simulink model "summer21"  (R2021a)
settings: Solver=VariableStepAuto  StartTime=0.0  StopTime=15  RelTol=1e-3
values from neighbouring files (symbols this model uses):
  C = num{1}(2:end)    [MR2007_final_P1_vt17.m]    (also in MR2007_final_fall17.m = [1, 0]; MR2007_final_p2.m = [1, 0]; MR2007_summer2021.m = B; map.m = [1, 0])
  Gamma = [1;0]    [MR2007_final_P1_vt17.m]    (also in MR2007_final_fall17.m = [1/omega0^2*(cosh(omega0*h) - 1); 1/omega0*sinh(omega0*h)]; MR2007_final_p2.m = [0.5;1]; MR2007_summer2021.m)
  l0 = 1/dcgain(sys_c)    [MR2007_summer2021.m]
  L_e = acker(Phi_e, Gamma_e, [pc, 0.5])    [MR2007_summer2021.m]
  Phi = cat(1, -den{1}(2:end), [1, 0])    [MR2007_final_P1_vt17.m]    (also in MR2007_final_fall17.m = [cosh(omega0*h), 1/omega0*sinh(omega0*h); MR2007_final_p2.m = [1 1; 0 1]; MR2007_summer2021.m = [-A(2:end); 1 0])
settings Model: Creator=kjartan  LastModifiedBy=kjartan

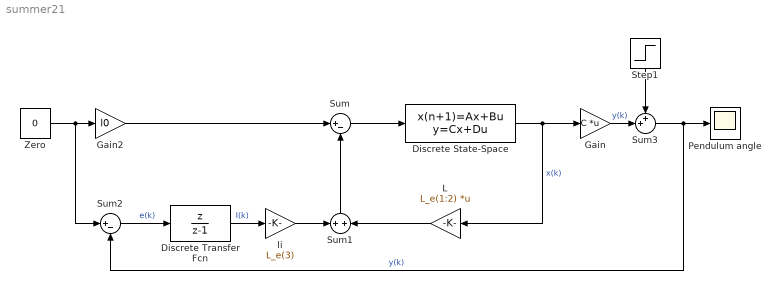
== system summer21 ==
  Discrete Transfer Fcn : DiscreteTransferFcn  Numerator=[1, 0]  Denominator=[1 -1]
  Discrete State-Space : DiscreteStateSpace  A=Phi  B=Gamma  C=eye(2)  D=zeros(2,1)  SampleTime=-1
  Gain : Gain  Gain=C  Multiplication=Matrix(K*u) (u vector)
  Gain2 : Gain  Gain=l0
  L : Gain  Gain=L_e(1:2)  Multiplication=Matrix(K*u) (u vector)
  Pendulum angle : Scope
  Step1 : Step  SampleTime=0
  Sum : Sum  Inputs=|+-
  Sum1 : Sum  Inputs=+|+
  Sum2 : Sum  Inputs=|+-
  Sum3 : Sum  Inputs=++|
  Zero : Constant  Value=0  OutDataTypeStr=Inherit: Inherit via back propagation
  li : Gain  Gain=L_e(3)
  wires:
  Discrete State-Space/1 -> L/1, Gain/1  "x(k)"
  Sum3/1 -> Sum2/2, Pendulum angle/1  "y(k)"
  Sum1/1 -> Sum/2
  L/1 -> Sum1/2
  Zero/1 -> Sum2/1, Gain2/1
  Sum2/1 -> Discrete Transfer Fcn/1  "e(k)"
  Discrete Transfer Fcn/1 -> li/1  "I(k)"
  li/1 -> Sum1/1
  Gain2/1 -> Sum/1
  Sum/1 -> Discrete State-Space/1
  Gain/1 -> Sum3/2  "y(k)"
  Step1/1 -> Sum3/1
